simulink model "TV_2017"  (R2016a)
settings: Solver=FixedStepAuto  StartTime=0.0  StopTime=inf  FixedStep=0.001  RelTol=1e-3
PreLoadFcn:
  | TV_2017_parameters
values from neighbouring files (symbols this model uses):
  battery_voltage = single(530)    [HIL_parameters.m]    (also in HIL_parameters_2018.m; TV_2017_parameters.m; TV_2017_parameters_VD.m)
  car_params = Simulink_Car_params    [HIL_parameters.m]    (also in HIL_parameters_2018.m; TV_2017_parameters.m; TV_2017_parameters_VD.m)
  i_Diff = 16    [HIL_parameters.m]    (also in HIL_parameters_2018.m; TV_2017_parameters.m)
  Kp = 1    [HIL_parameters.m]    (also in HIL_parameters_2018.m; TV_2017_parameters.m; TV_2017_parameters_VD.m)
  motor_data = struct    [HIL_parameters.m]    (also in HIL_parameters_2018.m; TV_2017_parameters.m)
  powerLimitControl = Simulink_el    [HIL_parameters.m]    (also in HIL_parameters_2018.m; TV_2017_parameters.m; TV_2017_parameters_VD.m)
  settings = Simulink_Settings    [HIL_parameters.m]    (also in HIL_parameters_2018.m; TV_2017_parameters.m; TV_2017_parameters_VD.m)
  SpdC_BCC = 0    [HIL_parameters.m]    (also in HIL_parameters_2018.m; TV_2017_parameters.m; TV_2017_parameters_VD.m)
  Speed_Neg_sat = -21    [HIL_parameters.m]    (also in HIL_parameters_2018.m; TV_2017_parameters.m; TV_2017_parameters_VD.m)
  Speed_Pos_sat = 21    [HIL_parameters.m]    (also in HIL_parameters_2018.m; TV_2017_parameters.m; TV_2017_parameters_VD.m)
  SteeringAngleFL = [-23.80 -22.65 -21.50 -20.34 -19.18 -18.03 -16.86 -15.70 -14.53 -13.35 -12.18 -10.99 -9.80 -8.61 -7.40 -6.19 -4.97 -3.75 -2.51 -1.26 0 1.27 2.56 3.85 5.17 6.50 7.84 9.21 10.59 12.00 13.42 14.88 16.36 17.87 19.41 20.99 22.61 24.26 25.97 27.73 29.54]    [CarSetupAnalysis2018.m]    (also in HIL_parameters_2018.m; TV_2017_parameters.m; TV_2017_parameters_VD.m = [-24.129 -22.950 -21.772 -20.593 -19.413 -18.232 -17.050 -15)
  SteeringAngleFR = [-29.54 -27.73 -25.97 -24.26 -22.61 -20.99 -19.41 -17.87 -16.36 -14.88 -13.42 -12.00 -10.59 -9.21 -7.84 -6.50 -5.17 -3.85 -2.56 -1.27 0 1.26 2.51 3.75 4.97 6.19 7.40 8.61 9.80 10.99 12.18 13.35 14.53 15.70 16.86 18.03 19.18 20.34 21.50 22.65 23.80]    [CarSetupAnalysis2018.m]    (also in HIL_parameters_2018.m; TV_2017_parameters.m; TV_2017_parameters_VD.m = [-29.3050 -27.5340 -25.8140 -24.1410 -22.5110 -20.9180 -19.3)
  SteeringWhAngle = [-105 -99.75 -94.5 -89.25 -84 -78.75 -73.5 -68.25 -63 -57.75 -52.5 -47.25 -42 -36.75 -31.5 -26.25 -21.0 -15.75 -10.5 -5.25 0.0 5.25 10.50 15.75 21.00 26.25 31.50 36.75 42.00 47.25 52.50 57.75  63.00 68.25 73.50 78.75 84.00 89.25 94.50 99.75 105.00]    [TV_2017_parameters_VD.m]
  Tn_n = 0    [HIL_parameters.m]    (also in HIL_parameters_2018.m; TV_2017_parameters.m; TV_2017_parameters_VD.m)
  tractionControl = Simulink_tc    [HIL_parameters.m]    (also in HIL_parameters_2018.m; IterativeTractionControlTuning.m; TV_2017_parameters.m; TV_2017_parameters_VD.m)
  yawMomentGenerator = struct    [HIL_parameters.m]    (also in HIL_parameters_2018.m = Simulink_yawRate2; TV_2017_parameters.m = Simulink_yawRate2)
  yawRateControl = Simulink_yawRate    [HIL_parameters.m]    (also in HIL_parameters_2018.m; TV_2017_parameters.m; TV_2017_parameters_VD.m)
undefined symbols (not defined in the file or in its folder): DiscIntNeverNeededParam, magnitude, speedEstimation, TC_Decr_Gas, TC_Derivative, TC_Incr_Gas, TC_On, TC_Relay_Off, TC_Relay_On
libraries: CarMaker4SL x350, simulink_extras x63, simulink x37, dspfdesign x2
(part 9 of 14)

== matlab function TV_2017/CarMaker/Control_System /Slip Rate Control /SMC Traction Control/MATLAB Function ==
  data: Ti_FL input; Ti_FR input; Ti_lim output Bus: Ti_lim; Ti_RL input; Ti_RR input; TC_FL input; TC_FR input; TC_RL input; TC_RR input; states input Bus: States; T_req input
function Ti_lim =  TCOutputHandling(Ti_FL, Ti_FR, Ti_RL, Ti_RR, TC_FL,TC_FR,TC_RL,TC_RR,states, T_req)
%#codegen

yawRate_p_lim = 0.2;
ay_p_lim = 3;

straightline = uint32(0);

if ( (states.r > -yawRate_p_lim) && (states.r < yawRate_p_lim) && ...
     (states.ay > -ay_p_lim) && (states.ay < ay_p_lim) )
    straightline = 1;
else
    straightline = 0;
end


% Proposal : TC only active if yaw rate within some set

% FRONT SIDE
n_cmp = single(-0.03);
p_cmp = single(0.03);

% If driving ~ straightline then couple the outputs
% Else, each TC works individually. 
if      ( (straightline == 1) && (T_req > p_cmp) )
    % Couple TC outputs to maintain stability on mu split surfaces 
    % under acceleration and deceleration
    Ti_lim.FL = max(0, (Ti_FL + min(TC_FL,TC_FR) ) );
    Ti_lim.FR = max(0, (Ti_FR + min(TC_FL,TC_FR) ) );
    
    Ti_lim.RL = max(0, (Ti_RL + min(TC_RL,TC_RR) ) );
    Ti_lim.RR = max(0, (Ti_RR + min(TC_RL,TC_RR) ) );
 
elseif  ( (straightline) && (T_req < n_cmp) )
    % Couple TC outputs to maintain stability on mu split surfaces 
    % under acceleration and deceleration
    Ti_lim.FL = min(0, (Ti_FL + max(TC_FL,TC_FR) ) );
    Ti_lim.FR = min(0, (Ti_FR + max(TC_FL,TC_FR) ) );
    
    Ti_lim.RL = min(0, (Ti_RL + max(TC_RL,TC_RR) ) );
    Ti_lim.RR = min(0, (Ti_RR + max(TC_RL,TC_RR) ) );   
else
    % Decouple TC outputs to avoid interferring too much with the stability
    % of the vehicle while cornering. This is the DYC systems job. 
    Ti_lim.FL = Ti_FL + TC_FL;
    Ti_lim.FR = Ti_FR + TC_FR;
    Ti_lim.RL = Ti_RL + TC_RL;
    Ti_lim.RR = Ti_RR + TC_RR;
end

end




% if      ( (TC_FL < n_cmp) && (TC_FR < n_cmp) )
%     % add the most negative
% elseif  ( (TC_FL > p_cmp) && (TC_FR > p_cmp) )
%     % Add the most positive
%     
% elseif  ( (TC_FL < n_cmp) && (TC_FR > p_cmp) )
%     % Individual control
% elseif  ( (TC_FL > p_cmp) && (TC_FR < n_cmp) )
%     % Individual control
%     
%     
% elseif  ( (TC_FL > p_cmp) && (TC_FR < p_cmp) && (TC_FR > n_cmp) && (T_req < n_cmp) )
%     % One wants to add, other is fine and T_req < 0 which means it must be
%     % braking either straight or into a corner.. Add to both wheels, but do
%     % not exceed 0 torque.
%     
% elseif  ( (TC_FL < p_cmp) && (TC_FL > n_cmp) && (TC_FR > p_cmp)  && (T_req < n_cmp) )
%     % One wants to add, other is fine and T_req < 0 which means it must be
%     % braking either straight or into a corner.. Add to both wheels, but do
%     % not exceed 0 torque.    
%     
% elseif  ( (TC_FL < n_cmp) && ( (TC_FR < p_cmp) && (TC_FR > n_cmp) ) ...
%           && (T_req > p_cmp) && (straightline))
%     % One wants to subtract, other is fine and T_req > 0 and straightline
%     % which means mu split acceleration.
%     
%  elseif  ( (TC_FL > n_cmp) && (TC_FL < p_cmp) && (TC_FR < n_cmp) ) ...
%           && (T_req > p_cmp) && (straightline))
%     % One wants to subtract, other is fine and T_req > 0 and straightline
%     % which means mu split acceleration.    
%     
% elseif  ( (TC_FL < n_cmp) &&  (TC_FR < p_cmp) && (TC_FR > n_cmp) ...
%            && (not(straightline)))
%     % One wants to subtract, other is fine and T_req > 0 and straightline
%     % is false which means
%     
%  elseif  ( (TC_FL > n_cmp) && (TC_FL < p_cmp) && (TC_FR < n_cmp)  ...
%            && (not(straightline)))
%     % One wants to subtract, other is fine and T_req > 0 and straightline
%     % which means mu split acceleration.       
% elseif  
%     
%     
% y = u;

== matlab function TV_2017/CarMaker/Control_System /Slip Rate Control /SMC Traction Control/MATLAB Function1 ==
  data: states input Bus: States; SR_FL output; SR_FR output; SR_RL output; SR_RR output; vx output
function [SR_FL,SR_FR,SR_RL,SR_RR,vx] = extractSlipRatios(states)
%#codegen


SR_FL = states.SR_FL;
SR_FR = states.SR_FR;
SR_RL = states.SR_RL;
SR_RR = states.SR_RR;

vx = states.V_x;

== matlab function TV_2017/CarMaker/Vehicle dynamics analysis/MATLAB Function ==
  data: Force input; MM output; Moment input; car_params parameter
function MM = MagicMumber(Force,Moment,car_params)
WB = car_params.l;              % Wheelbase
Lf = 2.03-car_params.AeroRefX;  % Distance from aero referance to front axle
Fz = Force(3);                  % aerodynamic lift
PM = Moment(2);                 % aerodynamic pitch moment
Fr = (-PM-Fz.*Lf)./WB;           % aerodynamic load rear axle
Ff = -Fz-Fr;                    % aerodynamic load front axle
MM = Fr./(Ff+Fr);               % front-rear aerodynamic balance metric

end

== matlab function TV_2017/CarMaker/Control_System /Slip Rate Control /SMC Traction Control/Slip Rate FL/SMC ==
  data: muOfSlip input; TC output; SR input; SR_ref input; car_params parameter; states input; K input
function TC = fcn(muOfSlip,SR,SR_ref,car_params, states,K)
%#codegen
Jr = 0.2;
GR = car_params.GR;
r = car_params.r_eff;
m = car_params.mass;
Fz_FL = states.Fz_FL;
%slip = ((Jr/(m*r^2*(1-SR))) +1 )*muOfSlip*Fz_FL*r

ySlip = (r*(1-SR)^2)/(Jr*states.V_x);
force = muOfSlip*Fz_FL*r/GR
TC = force - (K/(ySlip))*sign(SR-SR_ref)*min(1,abs(SR-SR_ref));

== matlab function TV_2017/CarMaker/Control_System /Slip Rate Control /SMC Traction Control/Slip Rate FL1/SMC ==
  data: muOfSlip input; TC output; SR input; SR_ref input; car_params parameter; states input; K input
function TC = fcn(muOfSlip,SR,SR_ref,car_params, states,K)
%#codegen
Jr = 0.2;
GR = car_params.GR;
r = car_params.r_eff;
m = car_params.mass;
Fz_FR = states.Fz_FR;
%slip = ((Jr/(m*r^2*(1-SR))) +1 )*muOfSlip*Fz_FL*r
ySlip = (r*(1-SR)^2)/(Jr*states.V_x);
force = muOfSlip*Fz_FR*r/GR
TC = force - (K/(ySlip))*sign(SR-SR_ref)*min(1,abs(SR-SR_ref));

== matlab function TV_2017/CarMaker/Control_System /Slip Rate Control /SMC Traction Control/Slip Rate FL2/SMC ==
  data: muOfSlip input; TC output; SR input; SR_ref input; car_params parameter; states input; K input
function TC = fcn(muOfSlip,SR,SR_ref,car_params, states,K)
%#codegen
Jr = 0.2;
GR = car_params.GR;
r = car_params.r_eff;
m = car_params.mass;
Fz_RL = states.Fz_RL;
%slip = ((Jr/(m*r^2*(1-SR))) +1 )*muOfSlip*Fz_FL*r
ySlip = (r*(1-SR)^2)/(Jr*states.V_x);
force = muOfSlip*Fz_RL*r/GR
TC = force - (K/(ySlip))*sign(SR-SR_ref)*min(1,abs(SR-SR_ref));

== matlab function TV_2017/CarMaker/Control_System /Slip Rate Control /SMC Traction Control/Slip Rate FL3/SMC ==
  data: muOfSlip input; TC output; SR input; SR_ref input; car_params parameter; states input; K input
function TC = fcn(muOfSlip,SR,SR_ref,car_params, states,K)
%#codegen
Jr = 0.2;
GR = car_params.GR;
r = car_params.r_eff;
m = car_params.mass;
Fz_RR = states.Fz_RR;
%slip = ((Jr/(m*r^2*(1-SR))) +1 )*muOfSlip*Fz_FL*r
ySlip = (r*(1-SR)^2)/(Jr*states.V_x);
force = muOfSlip*Fz_RR*r/GR
TC = force - (K/(ySlip))*sign(SR-SR_ref)*min(1,abs(SR-SR_ref));

== matlab function TV_2017/CarMaker/Estimations/calculateMeanWheelAngle/calculateWheelangleandSpeed ==
  data: mean_wheel_angle output single; sensor input Bus: SensorInputs; mean_wheel_speed output single
function [mean_wheel_angle, mean_wheel_speed] = calculateWheelAngle(sensor)
%#codegen

% Right now assumes rad for angle, and rad/s for speed
mean_wheel_angle    = single(0.2536*sensor.steering_wheel_angle);
mean_wheel_speed    = single(0.2536*sensor.steering_wheel_speed);

end

== matlab function TV_2017/CarMaker/Estimations/Fz_estimators/Fz_Estimation/FzEstDamper ==
  data: sensors input Bus: SensorInputs; Fz_damp_FL input; Fz_damp_FR input; Fz_damper_est output Bus: normalForces; Fz_damp_RL input; Fz_damp_RR input; car_params parameter; alfa_r output
function [Fz_damper_est, alfa_r] =  FzEstDamp(sensors, Fz_damp_FL, Fz_damp_FR, Fz_damp_RL, Fz_damp_RR, car_params)
%#codegen

Ks_front    = car_params.spring_constant_front;
Ks_rear     = car_params.spring_constant_rear;
unsprung_front = car_params.unsprung_mass_per_wheel_newton_front; 
unsprung_rear  = car_params.unsprung_mass_per_wheel_newton_rear; 
half_track_front =  car_params.t_f;
half_track_rear  =  car_params.t_r;
arb_Ks_front     = car_params.arb_f_Nm_rad;
arb_Ks_rear      = car_params.arb_r_Nm_rad;
damper_pos_FL = sensors.damper_pos_FL ;
damper_pos_FR = sensors.damper_pos_FR ;
damper_pos_RL = sensors.damper_pos_RL ;
damper_pos_RR = sensors.damper_pos_RR ;

FL_preload = car_params.preload_front_mm * Ks_front;% * 0.001;
FR_preload = car_params.preload_front_mm * Ks_front;% * 0.001;
RL_preload = car_params.preload_rear_mm * Ks_rear;% * 0.001;
RR_preload = car_params.preload_rear_mm * Ks_rear;% * 0.001;

%add unsprung mass to Fz estimate gradualy as spring compress (not during wheel lift )
add_unsprung_threshold = 2;
scale = 1 / add_unsprung_threshold;
FL_unsprung = single((unsprung_front+FL_preload) * scale *  max(   0,  min(    damper_pos_FL , single(add_unsprung_threshold)   )));
FR_unsprung = single((unsprung_front+FR_preload) * scale *  max(   0,  min(    damper_pos_FR , single(add_unsprung_threshold)   )));
RL_unsprung = single((unsprung_rear+RL_preload) * scale *  max(   0,  min(    damper_pos_RL , single(add_unsprung_threshold)   )));
RR_unsprung = single((unsprung_rear+RR_preload) * scale *  max(   0,  min(    damper_pos_RR , single(add_unsprung_threshold)   )));

%adjust estimate for ARB weight transfer

arb_transfer_f = arb_Ks_front * sensors.roll_angle * half_track_front; 
arb_transfer_r = arb_Ks_rear * sensors.roll_angle * half_track_rear; 
K_damp_front=800;
K_damp_rear =800;
%estimate forces from spring, damper and ARB
min_value = 100;
Fz_damper_est.FL = max(min_value ,  Ks_front*damper_pos_FL  + FL_unsprung);% - K_damp_front*Fz_damp_FL;%+ arb_transfer_f; % 
Fz_damper_est.FR = max(min_value ,  Ks_front*damper_pos_FR  + FR_unsprung);% - K_damp_front*Fz_damp_FR;%- arb_transfer_f; % 
Fz_damper_est.RL = max(min_value ,  Ks_rear*damper_pos_RL   + RL_unsprung);% - K_damp_rear*Fz_damp_RL;%+ arb_transfer_r; % 
Fz_damper_est.RR = max(min_value ,  Ks_rear*damper_pos_RR   + RR_unsprung);% - K_damp_rear*Fz_damp_RR;%- arb_transfer_r; % 

alfa_r = max(1,(Fz_damper_est.RL + Fz_damper_est.RR)) / max(1,(Fz_damper_est.FL + Fz_damper_est.FR + Fz_damper_est.RL + Fz_damper_est.RR));

== matlab function TV_2017/CarMaker/Control_System /Subsystem/Torque allocation 2016/Torque Allocation/TorqueAllocation ==
  data: Ti_lim output Bus: Ti_lim; T_req input; states input; maxMotorTorque input; settings parameter; car_params parameter; Mz_ref input; Ti_max output; Mz_error output; Mz_allocated output; yawRateControl parameter
function [Ti_lim,Ti_max,Mz_error, Mz_allocated]  = torqueAllocation(T_req,states,maxMotorTorque,settings, car_params, Mz_ref,yawRateControl)
%#codegen

%STATES
r = states.r;
negative_torque_limit = yawRateControl.negative_torque_limit;

%PARAMETERS
%mu = states.mu;
mu = settings.mu;
tf = car_params.t_f*2;
tr = car_params.t_r*2;
GR = car_params.GR;
r_eff = car_params.r_eff;
R = [r_eff; r_eff; r_eff; r_eff]';


Fzi = [max(1,states.Fz_FL) max(1,states.Fz_FR) max(1,states.Fz_RL) max(1,states.Fz_RR)]';
switch settings.TV_Method
    case 1
        % Only positive Torque
       alfa_r =  (Fzi(3) + Fzi(4)) / (Fzi(1) + Fzi(2) + Fzi(3) + Fzi(4));
    case 2
        % Can also allocate negative torque
       alfa_r =  (Fzi(3) + Fzi(4)) / (Fzi(1) + Fzi(2) + Fzi(3) + Fzi(4));
       %alfa_r = single(0.5)  test dette for å se om distribusjonen blir
       %lik ev soverestimer friksjonspotensialet
    case 3
        % Static 25 percent to each wheel
        alfa_r = single(0.5);
    case 4
        % Allocation with negative torque, but does not use Fz
        alfa_r = single(0.5); 
    otherwise
        alfa_r = single(0.5);       
end

S = states.wheel_angle;

l1 = car_params.t_f*cos(S);
l2 = car_params.t_f*cos(S);
l3 = car_params.t_r;
l4 = car_params.t_r;
L = [-l1; l2; -l3; l4];



%FIND MAXIMUM ALLOWED MOTOR TORQUE, TIRE/MOTOR
Ti_max          = single(zeros(4,1));
Ti_max_tire     = single(zeros(4,1));

RPM = [states.RPM_FL, states.RPM_FR, states.RPM_RL, states.RPM_RR];
Ti_max_motor = [maxMotorTorque.mmt_FL,maxMotorTorque.mmt_FR,maxMotorTorque.mmt_RL,maxMotorTorque.mmt_RR]; 

%Tire saturation based on mu and Fz
for i=1:4
    Ti_max_tire(i) = Fzi(i)*mu*R(i)/GR;
end

%Find minimum of tire saturation Torque and motor
for i=1:4
    Ti_max(i) = min(Ti_max_tire(i), Ti_max_motor(i));
end
%**********************************************%

T_F = single(zeros(2,1));
T_R = single(zeros(2,1));
sat_F = uint32(0);
sat_R = uint32(0);

if ( T_req >= 0)
    switch settings.TV_Method
        case 1
            % Only positive Torque
            [T_F, sat_F] = allocatePositiveTorque(Ti_max(1), Ti_max(2), T_req, R(1), R(2), (1-alfa_r), Mz_ref, GR, tf);
            [T_R, sat_R] = allocatePositiveTorque(Ti_max(3), Ti_max(4), T_req, R(3), R(4), alfa_r, Mz_ref, GR, tr);
        case 2
            % Can also allocate negative torque
            [T_F, sat_F] = allocateTorque(Ti_max(1), Ti_max(2), T_req, R(1), R(2), (1-alfa_r), Mz_ref, GR, tf, negative_torque_limit);
            [T_R, sat_R] = allocateTorque(Ti_max(3), Ti_max(4), T_req, R(3), R(4), alfa_r, Mz_ref, GR, tr ,negative_torque_limit);
        case 3
            % Static 25 percent to each wheel
            T_F = [0.25*T_req; 0.25*T_req];
            T_R = [0.25*T_req; 0.25*T_req];
        case 4
            % Allocation with negative torque, but does not use Fz
            [T_F, sat_F] = allocateTorque(Ti_max_motor(1), Ti_max_motor(2), T_req, R(1), R(2), (1-alfa_r), Mz_ref, GR, tf, negative_torque_limit);
            [T_R, sat_R] = allocateTorque(Ti_max_motor(3), Ti_max_motor(4), T_req, R(3), R(4), alfa_r, Mz_ref, GR, tr ,negative_torque_limit);
    end
            
    if ( (sat_F == 1) && (sat_R == 1) )
        % Nothing more to do
    elseif ( (sat_F == 1) && (sat_R == 0) )     
         if ( T_F(1) < 0) 
            T_remaining = T_req - (T_F(2));
         elseif (T_F(2) < 0) 
             T_remaining = T_req - (T_F(1));
         else
             T_remaining = T_req - (T_F(1) + T_F(2));
         end
         
         if (yawRateControl.enable == 1)
             Mz_remaining = Mz_ref - (-l1*GR*T_F(1)/R(1) + l2*GR*T_F(2)/R(2));
         else
             Mz_remaining = single(0);
         end 
         
        switch settings.TV_Method
            case 1
                % Only positive Torque
                [T_R sat_R] = allocatePositiveTorque(Ti_max(3), Ti_max(4), T_remaining, R(3), R(4), 1 , Mz_remaining, GR, tr);
            case 2
                % Can also allocate negative torque
                [T_R sat_R] = allocateTorque(Ti_max(3), Ti_max(4), T_remaining, R(3), R(4), 1 , Mz_remaining, GR, tr,negative_torque_limit);
            case 4
                [T_R sat_R] = allocateTorque(Ti_max_motor(3), Ti_max_motor(4), T_remaining, R(3), R(4), 1 , Mz_remaining, GR, tr,negative_torque_limit);
        end 
    elseif ( (sat_F == 0) && (sat_R == 1) )
         if ( T_R(1) < 0) 
            T_remaining = T_req - (T_R(2));
         elseif (T_R(2) < 0) 
             T_remaining = T_req - (T_R(1));
         else
             T_remaining = T_req - (T_R(1) + T_R(2));
         end        
        % For example rear is saturated, and front can still use more torque
        %T_remaining = T_req - (T_R(1) + T_R(2));
        if (yawRateControl.enable == 1)
             Mz_remaining = Mz_ref - (-l3*GR*T_R(1)/R(3) + l4*GR*T_R(2)/R(4));
        else
             Mz_remaining = single(0);
        end 
        %Mz_remaining = Mz_ref*(1-alfa_r);
        switch settings.TV_Method
            case 1
                % Only positive Torque
                 [T_F sat_F] = allocatePositiveTorque(Ti_max(1), Ti_max(2), T_remaining, R(1), R(2), 1 , Mz_remaining, GR, tf);
            case 2
                % Can also allocate negative torque
                [T_F sat_F] = allocateTorque(Ti_max(1), Ti_max(2), T_remaining, R(1), R(2), 1 , Mz_remaining, GR, tf,negative_torque_limit);
            case 4
                [T_F sat_F] = allocateTorque(Ti_max_motor(1), Ti_max_motor(2), T_remaining, R(1), R(2), 1 , Mz_remaining, GR, tf,negative_torque_limit);
        end      
    else
        %both false
        % Nothing to do here either
    end
else
    %REGENERATIVE BRAKE COMMAND ( T_DRIVER_REQ < 0 )
    switch settings.TV_Method
        case 1
            % Only positive Torque
            [T_F, sat_F] = allocateKersTorque(Ti_max(1), Ti_max(2), T_req, R(1), R(2), (1-alfa_r), Mz_ref, GR, tf);
            [T_R, sat_R] = allocateKersTorque(Ti_max(3), Ti_max(4), T_req, R(3), R(4), alfa_r, Mz_ref, GR, tr);
            
        case 2
            % Can also allocate negative torque
            [T_F, sat_F] = allocateKersTorque(Ti_max(1), Ti_max(2), T_req, R(1), R(2), (1-alfa_r), Mz_ref, GR, tf);
            [T_R, sat_R] = allocateKersTorque(Ti_max(3), Ti_max(4), T_req, R(3), R(4), alfa_r, Mz_ref, GR, tr);
        case 3
            % Static 25 percent to each wheel
            T_F = [0.25*T_req; 0.25*T_req];
            T_R = [0.25*T_req; 0.25*T_req];
        case 4
            % Allocation with negative torque, but does not use Fz
            [T_F, sat_F] = allocateKersTorque(Ti_max_motor(1), Ti_max_motor(2), T_req, R(1), R(2), (1-alfa_r), Mz_ref, GR, tf);
            [T_R, sat_R] = allocateKersTorque(Ti_max_motor(3), Ti_max_motor(4), T_req, R(3), R(4), alfa_r, Mz_ref, GR, tr);
    end
    if (sat_F == 1 && sat_R == 1)
        %Nothing more to do
        
    elseif (sat_F == 1 && sat_R == 0)
         T_remaining = T_req - (T_F(1) + T_F(2));
         %Disable Mz_remaining if yaw control disabled?
        if (yawRateControl.enable == 1)
             Mz_remaining = Mz_ref - (-l1*GR*T_F(1)/R(1) + l2*GR*T_F(2)/R(2));
        else
             Mz_remaining = single(0);
        end
        switch settings.TV_Method
            case 1
                % Only positive Torque
                [T_R sat_R] = allocateKersTorque(Ti_max(3), Ti_max(4), T_remaining, R(3), R(4), 1 , Mz_remaining, GR, tr);

            case 2
                % Can also allocate negative torque
                [T_R sat_R] = allocateKersTorque(Ti_max(3), Ti_max(4), T_remaining, R(3), R(4), 1 , Mz_remaining, GR, tr);
            case 3
                % Static 25 %
            case 4
                % Allocation with negative torque, but does not use Fz
                [T_R sat_R] = allocateKersTorque(Ti_max_motor(3), Ti_max_motor(4), T_remaining, R(3), R(4), 1 , Mz_remaining, GR, tr);
        end
        
    elseif (sat_F == 0 && sat_R == 1)
        %For example rear is saturated, and front can still use more torque
        T_remaining = T_req - (T_R(1) + T_R(2));
        %Mz_remaining = Mz_ref*(1-alfa_r);
        
        if (yawRateControl.enable == 1)
             Mz_remaining = Mz_ref - (-l3*GR*T_R(1)/R(3) + l4*GR*T_R(2)/R(4));
        else
             Mz_remaining = single(0);
        end
        switch settings.TV_Method
            case 1
                % Only positive Torque
                [T_F sat_F] = allocateKersTorque(Ti_max(1), Ti_max(2), T_remaining, R(1), R(2), 1 , Mz_remaining, GR, tf); 

            case 2
                % Can also allocate negative torque
                [T_F sat_F] = allocateKersTorque(Ti_max(1), Ti_max(2), T_remaining, R(1), R(2), 1 , Mz_remaining, GR, tf); 
            case 3
                % Static 25 %
            case 4
                % Allocation with negative torque, but does not use Fz
                [T_F sat_F] = allocateKersTorque(Ti_max_motor(1), Ti_max_motor(2), T_remaining, R(1), R(2), 1 , Mz_remaining, GR, tf);             
        end
    else
        %both false
        %Nothing to do here either
    end
end

Ti_all = [T_F' T_R'];

Ti_lim_struct = struct;
Ti_lim_struct.FL = Ti_all(1);
Ti_lim_struct.FR = Ti_all(2);
Ti_lim_struct.RL = Ti_all(3);
Ti_lim_struct.RR = Ti_all(4);

Ti_lim = Ti_lim_struct;

% Calculate what yaw moment that was achieved with the current 
% allocation
Fx_all = prod([Ti_all; 1./R;])*GR;
Mz_allocated = L'*Fx_all';
Mz_error = Mz_ref - Mz_allocated;
end


function [T, sat] = allocateTorque(L_max, R_max, T_req,...
          R_eff_L, R_eff_R, alfa, Mz_ref, GR, t, negative_torque_limit)
      
    T = single(zeros(2,1));
    sat = uint32(0);
    % Desired torque vectoring torque
    TV_des = abs(alfa*Mz_ref*R_eff_L/(GR*t)) + abs(alfa*Mz_ref*R_eff_R/(GR*t));
    % Take absolute value since T_req can be negative in case of KERS
    T_driver = alfa*T_req;

    if ( Mz_ref <= 0)
        % Implies that left side should realize the TV torque,
        % since only torque >= 0 is used here.
        % Mz is defined positive counter clockwise
        L = min( [TV_des, T_driver, L_max]); 
        if ( (L < TV_des) ) %&& (T_driver > 0))
            % Not fulfilled desired yaw moment
            R = - min( [(TV_des - L), R_max, negative_torque_limit]);
            T = [L;R];
        else
            max_t_add = min([(L_max-TV_des), R_max, (T_driver-L)/2]);
            L = L + max_t_add;
            R = max_t_add;
            T = [L;R];
        end
        % Floats comparison
        if ( (L + 0.001) < (T_driver))
            sat = uint32(1);
        end
        return;
    else
        R = min( [TV_des, T_driver, R_max]);
        %Max torque that can be added to both  
        if ( (R < TV_des) ) % && (T_driver > 0) )
            L = -min( [(TV_des - R), L_max,negative_torque_limit]);
            T = [L;R];
        else
            max_t_add = min([(R_max - TV_des),L_max, (T_driver-R)/2]);
            R = R + max_t_add;
            L = max_t_add;
            T = [L;R];
        end
        
        if ( (R + 0.001) < (T_driver))
            sat = uint32(1);
        end
        return;
    end
end

function [T, sat] = allocateKersTorque(L_max, R_max, T_req, R_eff_L, R_eff_R, alfa, Mz_ref, GR, t )
    T = single(zeros(2,1));
    sat = uint32(0);
    % Desired torque vectoring torque
    TV_des = abs(alfa*Mz_ref*R_eff_L/(GR*t)) + abs(alfa*Mz_ref*R_eff_R/(GR*t));
    % Take absolute value since T_req can be negative in case of KERS
    T_driver = abs(alfa*T_req);
   
    if (Mz_ref + 0.0001 >= 0)
        % Positive Mz_ref requires left side (inner wheels)
        % to brake more than the outer wheels.
        L = min( [TV_des, T_driver, L_max]);
        %Max torque that can be added to both
        if L_max < abs(TV_des)
            max_t_add = single(0);
        else
            max_t_add = min([(L_max-TV_des), R_max, (T_driver-L)/2]);
        end 
        L = - (L + max_t_add);
        R = - max_t_add;
        T = [L;R];
        % Floats comparison
        if ( (abs(L) + abs(R) + 0.001) < T_driver)
            sat = uint32(1);
        end
        return;
    else
        R = min( [abs(TV_des), T_driver, R_max]);
        %Max torque that can be added to both
        if R_max < abs(TV_des)
            max_t_add = single(0);
        else
            max_t_add = min([(R_max-abs(TV_des)), L_max, (T_driver-R)/2]);
        end
        R = - (R + max_t_add);
        L = - max_t_add;
        T = [L;R];
        % Floats comparison
        if ( (abs(L) + abs(R) + 0.001) < T_driver)
            sat = uint32(1);
        end
        return;
    end
end
function [T, sat] = allocatePositiveTorque(L_max, R_max, T_req,...
          R_eff_L, R_eff_R, alfa, Mz_ref, GR, t )
      
    T = single(zeros(2,1));
    sat = uint32(0);
    % Desired torque vectoring torque
    TV_des = abs(alfa*Mz_ref*R_eff_L/(GR*t)) + abs(alfa*Mz_ref*R_eff_R/(GR*t));
    % Take absolute value since T_req can be negative in case of KERS
    T_driver = alfa*T_req;

    if ( Mz_ref <= 0)
        % Implies that left side should realize the TV torque,
        % since only torque >= 0 is used here.
        % Mz is defined positive counter clockwise
        L = min( [TV_des, T_driver, L_max]);
        %Max torque that can be added to both
        %Skal det ikke være L < TV_des
        if L_max < abs(TV_des)
            max_t_add = single(0);
        else
            max_t_add = min([(L_max-TV_des), R_max, (T_driver-L)/2]);
        end 
        L = L + max_t_add;
        R = max_t_add;
        T = [L;R];  
        % Floats comparison
        if ( (L + R + 0.001) < (T_driver))
            sat = uint32(1);
        end
        return;
    else
        R = min( [abs(TV_des), T_driver, R_max]);
        %Max torque that can be added to both
        if R_max < abs(TV_des)
            max_t_add = single(0);
        else
            max_t_add = min([(R_max-abs(TV_des)),L_max, (T_driver-R)/2]);
        end
        R = R + max_t_add;
        L = max_t_add;
        T = [L;R];
        % Floats comparison
        if ( (L + R + 0.001) < (T_driver))
            sat = uint32(1);
        end
        return;
    end
end

== matlab function TV_2017/CarMaker/Estimations/1st_deriv/Diff_Function ==
  data: y_old output; y_old input; sensors input; y output; delta_t input; RPM_der output
function [y_old,y , RPM_der] = innerFunction(y_old, sensors, delta_t)

y_old = single(circshift(y_old,1));
y_old(1) = sensors.RPM_FL;
        
RPM_der = single(sensors.RPM_der_FL);

M = length(y_old);
N = 3;
nu = 1;
j = 1;

k = 1:M;

x = phi(M,N,nu,j,k,delta_t) .* y_old;

y = single(sum(x));

end

function p = phi(M,N,nu,j,k,delta_t)

fac = (factorial(N + j + nu + 1) .*...
    factorial(N + 1)) ./...
    (M .* delta_t) .^ j;

[i,k2,k1,k] = ndgrid(0:nu + N,0:j,0:N-j,k);

eliminator = i > nu + k1 + k2;

evalIn = inPhi(M,N,nu,j,k,i,k1,k2);
evalIn(eliminator) = 0;

p = fac * sum(sum(sum(evalIn)));

p = p(:);

end

function p = inPhi(M,N,nu,j,k,i,k1,k2)

p = ((-1).^(N + i - k1 - k2) .*...
    ((k./M).^(N + i - k1 - k2 + 1) - ...
    ((k-1)./M).^(N + i - k1 - k2 + 1)))./...
    (factorial(k1) .* factorial(k2) .* factorial(i).*...
    factorial(N - j - k1) .*...
    factorial(j - k2) .*...
    factorial(N - k1 - k2) .*...
    factorial(nu - i + k1 + k2) .*...
    (N - k1 + 1) .*...
    (N + i -k1 - k2 + 1));

end

function n = factorial(n)

fac = [1;1;2;6;24;120;720;5040;40320;362880;3628800;39916800;479001600;6227020800.00000;87178291200.0000;1307674368000.00;20922789888000.0;355687428096000;6.40237370572800e+15;1.21645100408832e+17;2.43290200817664e+18;5.10909421717094e+19;1.12400072777761e+21;2.58520167388850e+22;6.20448401733239e+23;1.55112100433310e+25;4.03291461126606e+26;1.08888694504184e+28;3.04888344611714e+29;8.84176199373970e+30;2.65252859812191e+32;8.22283865417792e+33;2.63130836933694e+35;8.68331761881189e+36;2.95232799039604e+38;1.03331479663861e+40;3.71993326789901e+41;1.37637530912263e+43;5.23022617466601e+44;2.03978820811974e+46;8.15915283247898e+47;3.34525266131638e+49;1.40500611775288e+51;6.04152630633738e+52;2.65827157478845e+54;1.19622220865480e+56;5.50262215981209e+57;2.58623241511168e+59;1.24139155925361e+61;6.08281864034268e+62;3.04140932017134e+64];
n(n<0) = 0;
n = fac(n + 1);

end

== matlab function TV_2017/CarMaker/Debug Information /Vehicle dynamics analysis JMH/MATLAB Function1 ==
  data: Force input; MM output; Moment input; car_params parameter
function MM = MagicMumber(Force,Moment,car_params)
WB = car_params.l;              % Wheelbase
Lf = 2.03-car_params.AeroRefX;  % Distance from aero referance to front axle
Fz = Force(3);                  % aerodynamic lift
PM = Moment(2);                 % aerodynamic pitch moment
Fr = (-PM-Fz.*Lf)./WB;           % aerodynamic load rear axle
Ff = -Fz-Fr;                    % aerodynamic load front axle
MM = Fr./(Ff+Fr);               % front-rear aerodynamic balance metric
end

== matlab function TV_2017/CarMaker/Debug Information /Vehicle dynamics analysis JMH/MATLAB Function ==
  data: V input; OM_transient output; Delta input; Ay input; YawRate input; car_params parameter; OM_steadystate output
function [OM_transient,OM_steadystate] = OversteerMetric(V,Delta,Ay,YawRate,car_params)
W = car_params.l;
avgDelta = mean(Delta).*pi/180;     
AKR = V.*tan(avgDelta)./W;
OM_transient = YawRate-AKR;
OM_steadystate = (Ay.*W)./V.^2-avgDelta;
end

== matlab function TV_2017/CarMaker/IPG Vehicle3/CarAndTrailer/Forces/Vehicle Forces/Aero R18 prelim/MATLAB Function ==
  data: Fx output; Vx input; Vy input; Fy output; Fz output; Mx output; My output; Mz output; coeffs input; car_params parameter
function [Fx,Fy,Fz,Mx,My,Mz] = AeroForceCalc(Vx,Vy,coeffs, car_params)
rho = double(car_params.AirDens);
A = double(car_params.aero_ref_area);
l = double(car_params.l);                % Wheelbase

V = sqrt(Vx^2+Vy^2);

Cd = coeffs(1);
Cs = coeffs(2);
Cl = coeffs(3);
Crm = coeffs(4);
Cpm = coeffs(5);
Cym = coeffs(6);

Fx = -(rho/2)*Cd*A*V^2;     % Drag force
Fy = (rho/2)*Cs*A*V^2;     % Side force
Fz = -(rho/2)*Cl*A*V^2;     % Downforce
Mx = (rho/2)*Crm*l*A*V^2;   % Roll moment
My = (rho/2)*Cpm*l*A*V^2;   % Pitch moment
Mz = (rho/2)*Cym*l*A*V^2;   % Yaw moment


end

== matlab function TV_2017/CarMaker/Control_System /Power Limit Torque Reduction Controller 2018/Motorestimates/extractPower2 ==
  data: T_FL output; states input; RPM_FL output; T_FR output; RPM_FR output; T_RL output; RPM_RL output; T_RR output; RPM_RR output; Ti_lim input
function [T_FL, RPM_FL, T_FR, RPM_FR, T_RL, RPM_RL, T_RR, RPM_RR]= extractRPM(states, Ti_lim)
%#codegen
RPM_FL = states.RPM_FL;
RPM_FR = states.RPM_FR;
RPM_RL = states.RPM_RL;
RPM_RR = states.RPM_RR;

T_FL = Ti_lim.FL;
T_FR = Ti_lim.FR;
T_RL = Ti_lim.RL;
T_RR = Ti_lim.RR;

end

== matlab function TV_2017/CarMaker/Debug Information /Fz_Estimation/FzEstDamper ==
  data: sensors input Bus: SensorInputs; Fz_damp_FL input; Fz_damp_FR input; Fz_damper_est output Bus: normalForces; Fz_damp_RL input; Fz_damp_RR input; car_params parameter; alfa_r output
function [Fz_damper_est, alfa_r] =  FzEstDamp(sensors, Fz_damp_FL, Fz_damp_FR, Fz_damp_RL, Fz_damp_RR, car_params)
%#codegen

Ks_front    = car_params.spring_constant_front;
Ks_rear     = car_params.spring_constant_rear;

 

preload_front = car_params.preload_front_mm;
preload_rear = car_params.preload_rear_mm;

unsprung = car_params.unsprung_mass_per_wheel_newton;

%esimate forces from spring and damper

Fz_damper_est.FL = Ks_front*sensors.damper_pos_FL + Fz_damp_FL;% 
Fz_damper_est.FR = Ks_front*sensors.damper_pos_FR + Fz_damp_FR;% 
Fz_damper_est.RL = Ks_rear*sensors.damper_pos_RL + Fz_damp_RL;% 
Fz_damper_est.RR = Ks_rear*sensors.damper_pos_RR + Fz_damp_RR;% 

alfa_r = (Fz_damper_est.RL + Fz_damper_est.RR) / (Fz_damper_est.FL + Fz_damper_est.FR + Fz_damper_est.RL + Fz_damper_est.RR);

%add unsprung mass to Fz estimate only when spring is loaded
add_unsprung_threshold = 10;
if (Fz_damper_est.FL>add_unsprung_threshold)
    Fz_damper_est.FL = Fz_damper_est.FL + unsprung; 
end
if (Fz_damper_est.FR>add_unsprung_threshold)
    Fz_damper_est.FR = Fz_damper_est.FR + unsprung; 
end
if (Fz_damper_est.RL>add_unsprung_threshold)
    Fz_damper_est.RL = Fz_damper_est.RL + unsprung; 
end
if (Fz_damper_est.RR>add_unsprung_threshold)
    Fz_damper_est.RR = Fz_damper_est.RR + unsprung; 
end


end

== matlab function TV_2017/CarMaker/Debug Information /Fz_Estimation/FzEstDamper 2016 ==
  data: sensors input Bus: SensorInputs; Fz_damp_FL input; Fz_damp_FR input; Fz_damper_est output Bus: normalForces; Fz_damp_RL input; Fz_damp_RR input; car_params parameter; alfa_r output
function [Fz_damper_est, alfa_r] =  FzEstDamp(sensors, Fz_damp_FL, Fz_damp_FR, Fz_damp_RL, Fz_damp_RR, car_params)
%#codegen

Ks_front    = car_params.spring_constant_front;
Ks_rear     = car_params.spring_constant_rear;

MR_front    = car_params.motion_ratio_front;
MR_rear     = car_params.motion_ratio_rear;     

preload_front = car_params.preload_front_mm;
preload_rear = car_params.preload_rear_mm;

%unsprung = car_params.unsprung_mass_per_wheel_newton;
% 0 - 1 mm, Go from 0 to neutral Fz
FL_scaling = single(min(sensors.damper_pos_FL, single(1)));
FR_scaling = single(min(sensors.damper_pos_FR, single(1)));
RL_scaling = single(min(sensors.damper_pos_RL, single(1)));
RR_scaling = single(min(sensors.damper_pos_RR, single(1)));

% Fz_damper_est.FL = (Ks_front*(sensors.damper_pos_FL + preload_front) + Fz_damp_FL)*MR_front + unsprung;
% Fz_damper_est.FR = (Ks_front*(sensors.damper_pos_FR + preload_front) + Fz_damp_FR)*MR_front + unsprung;
% Fz_damper_est.RL = (Ks_rear*(sensors.damper_pos_RL  + preload_rear)  + Fz_damp_RL)*MR_rear  + unsprung;
% Fz_damper_est.RR = (Ks_rear*(sensors.damper_pos_RR  + preload_rear)  + Fz_damp_RR)*MR_rear  + unsprung;

Fz_damper_est.FL = Ks_front*sensors.damper_pos_FL + Fz_damp_FL + (preload_front*Ks_front)*FL_scaling;
Fz_damper_est.FR = Ks_front*sensors.damper_pos_FR + Fz_damp_FR + (preload_front*Ks_front)*FR_scaling;
Fz_damper_est.RL = Ks_rear*sensors.damper_pos_RL + Fz_damp_RL + (preload_rear*Ks_rear)*RL_scaling;
Fz_damper_est.RR = Ks_rear*sensors.damper_pos_RR + Fz_damp_RR + (preload_rear*Ks_rear)*RR_scaling;

alfa_r = (Fz_damper_est.RL + Fz_damper_est.RR) / (Fz_damper_est.FL + Fz_damper_est.FR + Fz_damper_est.RL + Fz_damper_est.RR);
end

== matlab function TV_2017/CarMaker/Debug Information /Fz_Estimation/FzEstLoadTransfer ==
  data: Fz_loadTransfer_est output Bus: normalForces; sensor input Bus: SensorInputs; car_params parameter; vx input
function Fz_loadTransfer_est  = FzEstLoadTransfer(sensor,car_params,vx)
%#codegen




mv = car_params.car_mass + car_params.driver_mass; % Total mass( driver + car) X
l  = car_params.l; %Wheel base X
lr = car_params.l_r; % X
lf = car_params.l_f;% X

ef = car_params.t_f*2; % Front track X
er = car_params.t_r*2; % Rear track X


hc = car_params.CoG_height; % X
g = 9.81; % X
air_density = single(1.2);

Fz_loadTransfer_est.FL = single(0);%(0.5*mv*(lr*g/l - hc*sensor.ax/l) - mv*(lr*g/l - hc*sensor.ax/l)*hc*sensor.ay/(ef*g))  + (vx^2 * car_params.aero_ref_area* car_params.aero_lift_coeff*air_density)/8;
Fz_loadTransfer_est.FR = single(0);%(0.5*mv*(lr*g/l - hc*sensor.ax/l) + mv*(lr*g/l - hc*sensor.ax/l)*hc*sensor.ay/(ef*g))  + (vx^2 * car_params.aero_ref_area* car_params.aero_lift_coeff*air_density)/8;
Fz_loadTransfer_est.RL = single(0);%(0.5*mv*(lf*g/l + hc*sensor.ax/l) - mv*(lf*g/l + hc*sensor.ax/l)*hc*sensor.ay/(er*g))  + (vx^2 * car_params.aero_ref_area* car_params.aero_lift_coeff*air_density)/8;
Fz_loadTransfer_est.RR = single(0);%(0.5*mv*(lf*g/l + hc*sensor.ax/l) + mv*(lf*g/l + hc*sensor.ax/l)*hc*sensor.ay/(er*g))  + (vx^2 * car_params.aero_ref_area* car_params.aero_lift_coeff*air_density)/8;

end

== matlab function TV_2017/CarMaker/Debug Information /Subsystem/MATLAB Function ==
  data: RPM_FL_IN input; RPM_FR_IN input; RPM_RL_IN input; RPM_RR_IN input; Pm_FL output; T input; T_FL output; RPM_FL output; Pm_FR output; T_FR output; RPM_FR output; Pm_RL output; T_RL output; RPM_RL output; Pm_RR output; T_RR output; RPM_RR output
function [Pm_FL, T_FL, RPM_FL,Pm_FR, T_FR, RPM_FR,Pm_RL, T_RL,...
          RPM_RL,Pm_RR, T_RR, RPM_RR] = powerMeasurement(RPM_FL_IN, RPM_FR_IN,RPM_RL_IN,RPM_RR_IN, T)
%#codegen

%Conversion from RPM to rad/s
c = single(2*pi/60);

T_FL = T.FL;
T_FR = T.FR;
T_RL = T.RL;
T_RR = T.RR;

RPM_FL = RPM_FL_IN;
RPM_FR = RPM_FR_IN;
RPM_RL = RPM_RL_IN;
RPM_RR = RPM_RR_IN;


Pm_FL = RPM_FL*c*T.FL;
Pm_FR = RPM_FR*c*T.FR;
Pm_RL = RPM_RL*c*T.RL;
Pm_RR = RPM_RR*c*T.RR;

== matlab function TV_2017/CarMaker/Control_System /Subsystem/Torque allocation 2017/Motor temperature limiter ==
  data: states input; maxMotorTorque output Bus: maxMotorTorque; settings parameter; car_params parameter
function maxMotorTorque = maxMotorTorque_MotorTemp(states,settings, car_params)
%#codegen

% The inverters limits output torque based on internal temperature
mmt = single(settings.max_motor_torque);
upper_max_temp = single(car_params.AMK_motor_upper_max_temp);
cutoff_temp    = single(car_params.AMK_motor_cutoff_temp);
torque = [mmt mmt 0]; %breakpoints for lookup function
temp = [0 upper_max_temp cutoff_temp];


mot_FL_temp = single(states.AMK_inverter_temp_FL);
mot_FR_temp = single(states.AMK_inverter_temp_RL);
mot_RL_temp = single(states.AMK_inverter_temp_RL);
mot_RR_temp = single(states.AMK_inverter_temp_RR);

%  y = interp1(xdata,ydata,x)
maxMotorTorque.mmt_FL = interp1(temp,torque,  mot_FL_temp  );
maxMotorTorque.mmt_FR = interp1(temp,torque,  mot_FR_temp  );
maxMotorTorque.mmt_RL = interp1(temp,torque,  mot_RL_temp  );
maxMotorTorque.mmt_RR = interp1(temp,torque,  mot_RR_temp  );

== matlab function TV_2017/CarMaker/Control_System /Subsystem/2016 adapted/MATLAB Function ==
  data: states input; maxMotorTorque output Bus: maxMotorTorque; settings parameter
function maxMotorTorque = findMaxMotorTorque(states,settings)
%#codegen

% DC Voltage                             / states
% Max allowable current draw in total    /settings
% Load distribution                      /states

Fzi = [max(1,states.Fz_FL) max(1,states.Fz_FR) max(1,states.Fz_RL) max(1,states.Fz_RR)]';

switch settings.TV_Method
    case 1 % No negative torque
        alfa_r =  (Fzi(3) + Fzi(4)) / (Fzi(1) + Fzi(2) + Fzi(3) + Fzi(4));
    case 2 % with negative torque
        alfa_r =  (Fzi(3) + Fzi(4)) / (Fzi(1) + Fzi(2) + Fzi(3) + Fzi(4));
    case 3 % static 25 %
        alfa_r = single(0.5);
    case 4 % with negative torque, no Fz
        alfa_r = single(0.5);
    otherwise
        alfa_r = single(0.5);
end

RPM_to_angular = single(2*pi/60);
omega_FL = states.RPM_FL*RPM_to_angular;
omega_FR = states.RPM_FR*RPM_to_angular;
omega_RL = states.RPM_RL*RPM_to_angular;
omega_RR = states.RPM_RR*RPM_to_angular;

mmt = settings.max_motor_torque;
available_power = states.DC_voltage*settings.max_battery_discharge;

max_torque_front = min(mmt, (available_power*(1-alfa_r))/ (2 * max( max(1,omega_FL), max(1,omega_FR))) );
max_torque_rear = min(mmt, (available_power*alfa_r)     / (2 * max( max(1,omega_RL), max(1,omega_RR))) );
                      
maxMotorTorque.mmt_FL = max_torque_front;
maxMotorTorque.mmt_FR = max_torque_front;
maxMotorTorque.mmt_RL = max_torque_rear;
maxMotorTorque.mmt_RR = max_torque_rear;
